simulink model "J2N6S200_simulink_Joint_manipulator"  (R2024a)
settings: Solver=VariableStepAuto  StartTime=0.0  StopTime=2  RelTol=1e-3
undefined symbols (not defined in the file): Sim3dSensor
libraries: sim3dlib x3, vrlib x3, robotcorelib x2, robotmaniplib x2, sim3dcameralib x2, visionsinks x2, robotsim3dlib x1, pycoexlib x1, dspvision x1
settings Model: Creator=abiro  LastModifiedBy=abiro

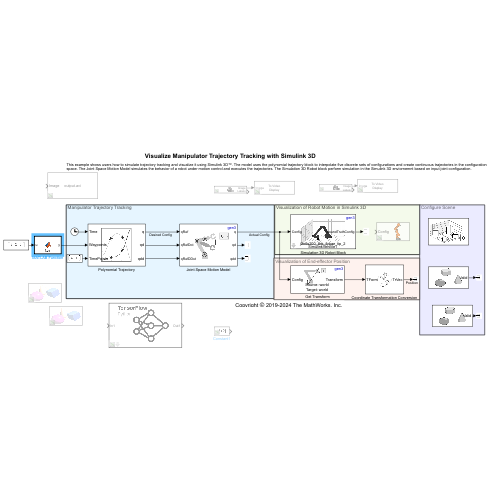
[thumbnail: Simulink's stored preview of the top-level diagram]
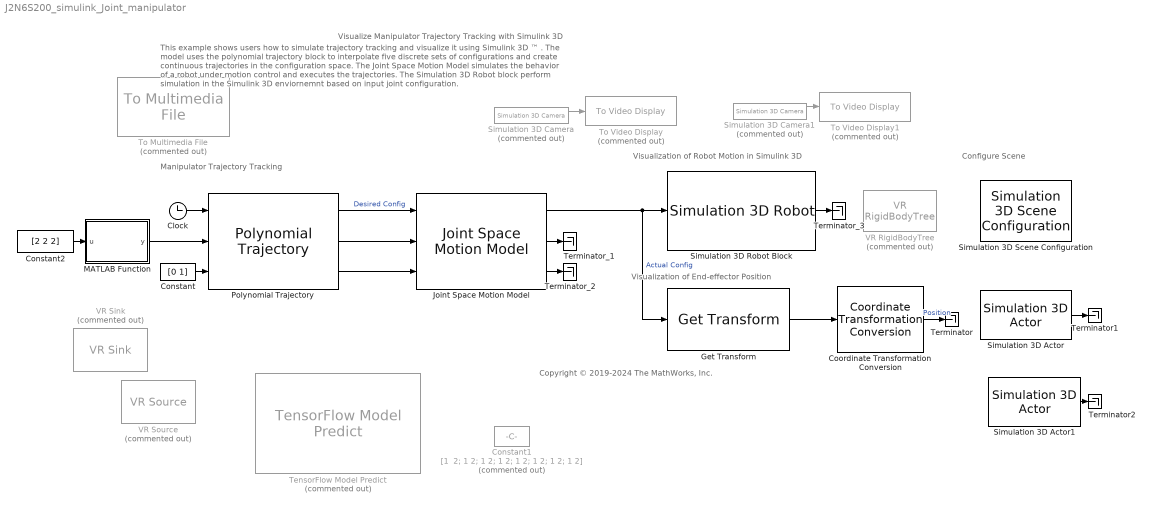
== system J2N6S200_simulink_Joint_manipulator ==
  note: Visualize Manipulator Trajectory Tracking with Simulink 3D
  note: Visualization of Robot Motion in Simulink 3D
  note: This example shows users how to simulate trajectory tracking and visualize it using Simulink 3D ™ . The model uses the polynomial trajectory block to interpolate five discrete sets of configurations and create continuous trajectories in the configuration space. The Joint Space Motion Model simulates the behavior of a robot under motion control and executes the trajectories. The Simulation 3D Robot block perform simulation in the Simulink 3D enviornemnt based on input joint configuration.
  note: Configure Scene
  note: Copyright © 2019-2024 The MathWorks, Inc.
  note: Visualization of End-effector Position
  note: Manipulator Trajectory Tracking
  Clock : Clock
  Constant : Constant  Value=[0 1]  VectorParams1D=off
  Constant1 : Constant  Commented=on  Value="[1  2; 1 2; 1 2; 1 2; 1 2; 1 2; 1 2; 1 2]"  VectorParams1D=off
  Constant2 : Constant  Value=[2 2 2]  VectorParams1D=off
  Coordinate Transformation Conversion : robotcorelib/Coordinate Transformation Conversion  InputRepresentation=Homogeneous Transformation  InputEulerSequence=ZYX  ShowTrVecInputPort=on  OutputRepresentation=Translation Vector  OutputEulerSequence=ZYX  ShowTrVecOutputPort=on  SimulateUsing=Interpreted execution
  Get Transform : robotmaniplib/Get Transform  RigidBodyTree=gen3  SourceBody=world  TargetBody=world  SimulateUsing=Interpreted execution
  Joint Space Motion Model : robotmaniplib/Joint Space Motion Model  RigidBodyTree=gen3  MotionType=Computed Torque Control  ProportionalGain=100  DerivativeGain=10  ErrorDynamicsSpecification=Damping Ratio / Natural Frequency  DampingRatio=1  NaturalFrequency=10  SettlingTime=0.59  Overshoot=0  ShowExternalForcePort=off  InitConfig=0  InitJointVel=0  SimulateUsing=Interpreted execution
  MATLAB Function : MATLAB Function  TreatAsAtomicUnit=on
  Polynomial Trajectory : robotcorelib/Polynomial Trajectory  WaypointSource=External  Waypoints=.75*pi*rand(8,2) - .375*pi  TimePoints=[ 0, 1]  TimeInterval=[ 1, 4 ]  Method=Cubic Polynomial  ParameterSource=Internal  VelocityBoundaryCondition=zeros( 8, 2 )  AccelerationBoundaryCondition=zeros( 2, 5 )  SimulateUsing=Interpreted execution
  Simulation 3D Actor : sim3dlib/Simulation 3D Actor  Priority=1  ActorName=Sim3dActor1  ParentName=Scene Origin  Operation=Create at setup  InitScriptText=|  SampleTime=-1  Translation=single([0 0 0])  Rotation=single([0 0 0])  Scale=single([1 1 1])  aMode=5  ActorTag=Sim3dActor1  ActorType=Sim3dActor  ID=1
      | % Reserved keywords:
      | % - Actor : handle to this actor object
      | % - World : handle to the world object
      | 
      | % Examples:
      | 
      | % Create a primitive geometry (optional)
      | Actor.createShape('box', [10 10 0.1]);
      | 
      | % Initialize values (optional)
      | Actor.Scale = 1;
      | Actor.Color = [0.2 0.2 0.2];
  Simulation 3D Actor1 : sim3dlib/Simulation 3D Actor  Priority=1  ActorName=Sim3dActor2  ParentName=Scene Origin  Operation=Create at setup  InitScriptText=|  SampleTime=-1  Translation=single([0 1 2])  Rotation=single([0 0 0])  Scale=single([1 1 1])  aMode=5  ActorTag=Sim3dActor2  ActorType=Sim3dActor  ID=2
      | % Reserved keywords:
      | % - Actor : handle to this actor object
      | % - World : handle to the world object
      | 
      | % Examples:
      | 
      | % Create a primitive geometry (optional)
      | Actor.createShape('box', [0.2 0.2 0.2]);
      | 
      | % Initialize values (optional)
      | Actor.Scale = 1;
      | Actor.Color = [0.2 0.2 0.2];
  Simulation 3D Camera : sim3dcameralib/Simulation 3D Camera  Priority=1  Commented=on  sensorTag=Sim3dSensor�  sensorId=1  sensorName=Sim3dSensor�  vehTagList={'Scene Origin';'Sim3dActor1';'SimulinkVehicle1'}  vehTag=Sim3dActor1  mountLoc=Origin  offsetFlag=on  tmountOffset=[-3.5, -1, 1]  extTmount=off  rmountOffset=[0, 0, 0]  extRmount=off  FocalLength=[1109, 1109]  OpticalCenter=[640, 360]  ImageSize=[720, 1280]  RadialDistortion=[0, 0]  TangentialDistortion=[0, 0]  SensorSkew=0  DepthOutportEnabled=off  SemanticOutportEnabled=on  TransformOutportEnabled=off  SampleTime=-1  mountPoint=[-3.5 1 1]  mountOrientation=[0 0 0]  aMode=6  ID=1
      settings: LibrarySourceBlock=robotsim3dlib/Simulation 3D Camera
  Simulation 3D Camera1 : sim3dcameralib/Simulation 3D Camera  Priority=1  Commented=on  sensorTag=Sim3dSensor�  sensorId=2  sensorName=Sim3dSensor�  vehTagList={'Scene Origin';'Sim3dActor1';'SimulinkVehicle1'}  vehTag=Sim3dActor1  mountLoc=Origin  offsetFlag=on  tmountOffset=[-3.5, 1, 1]  extTmount=off  rmountOffset=[0, 0, 0]  extRmount=off  FocalLength=[1109, 1109]  OpticalCenter=[640, 360]  ImageSize=[720, 1280]  RadialDistortion=[0, 0]  TangentialDistortion=[0, 0]  SensorSkew=0  DepthOutportEnabled=off  SemanticOutportEnabled=on  TransformOutportEnabled=off  SampleTime=-1  mountPoint=[-3.5 -1 1]  mountOrientation=[0 0 0]  aMode=6  ID=2
      settings: LibrarySourceBlock=robotsim3dlib/Simulation 3D Camera
  Simulation 3D Robot Block : robotsim3dlib/Simulation 3D Robot  actorInputType=RigidBodyTree Object  RigidBodyTree=gen3  ActorName=SimulinkVehicle1  existActorChekBox=off  initialTrans=[0 0 0]  initialRot=[0 0 0]  initialConfig="[0      3.1416      3.1416           0           0           0           0           0]"  EndEffector=j2n6s200_link_finger_tip_2  eeOffsetInpChekBox=off  eeTargetTrans=[0 0 0]  eeTargetRot=[0 0 0]  enableRegionGraspChekBox=off  regionGraspInpChekBox=off  eeTargTransDiff=[0.2 0.2 0.2]  eeTargRotDiff=[0 0 0]  inpConfEnbVal=on  inpGraspEnbVal=off  inpTransEnbVal=off  outConfEnbVal=on  outGraspEnbVal=off  outTransEnbVal=off  SampleTime=0.02  ActorType=SimulinkVehicle  ID=1  aMode=6  ActorTag=SimulinkVehicle1  Mesh=RigidBodyTree
  Simulation 3D Scene Configuration : sim3dlib/Simulation 3D Scene Configuration  Priority=0  ProjectFormat=Default Scenes  SceneDesc=Empty scene  ProjectName=C:\Program Files\MATLAB\R2024a\toolbox\shared\sim3d_projects\automotive_project_windows\UE\WindowsNoEditor\VehicleSimulation.exe  ScenePath=/Game/Maps/EmptyScene  EnableOpenDRIVE=off  vehTagList={'Custom';'Scene Origin';'Sim3dActor1';'SimulinkVehicle1'}  vehTag=Scene Origin  FreeCameraInitialTranslation=[0, 0, 0]  FreeCameraDefaultInitialTranslation=[-6, 0, 2]  FreeCameraInitialRotation=[0, 0, 0]  FreeCameraDefaultInitialRotation=[0, -15, 0]  OpVisEn=off  Ts=0.02  EnableWindow=on  EnableRemoteAccess=off  EnableWeather=off  SunAzimuth=90  SunAltitude=40.0  EnableGeospatialSun=off  Latitude=0  Longitude=0  Date=2023-01-01  Time=10:30:00  GeoTimeZone=-5.0  SunDaylightSaving=off  wind=1  clouds=10  EnableVolumetricClouds=off  CloudCoverage=0  CloudAltitude=6  fog=0  rain=0  RaindropsEffect=off  SnowDensity=0  EnableGeospatial=off  UseTrueOrigin=off  OriginHeight=200  OriginLatitude=40.744652  OriginLongitude=-73.988864  MapStyle=Aerial  AdditionalAssetIDs=[]  UseAdvancedSunSky=off  SolarTime=11  TimeZone=-5  Day=21  Month=9  Year=2022  UseDaylightSavingTime=on  DSTStartDay=10  DSTStartMonth=3  DSTEndDay=3  DSTEndMonth=11  DSTSwitchHour=2  sensorTag=MainCamera1  sensorId=1  sensorName=MainCamera1  mountLoc=Origin  offsetFlag=off  tmountOffset=[0, 0, 0]  rmountOffset=[0, 0, 0]  HorizontalResolution=1280  VerticalResolution=720  HorizontalFOV=60  mountPoint=[0 0 0]  mountOrientation=[0 0 0]  aMode=6  ID=1  GeoTrigger=Inactive
      settings: LibrarySourceBlock=robotsim3dlib/Simulation 3D Scene Configuration
  TensorFlow Model Predict : pycoexlib/TensorFlow Model Predict  Commented=on  ModelFile=untitled  InputTable={'In1','float32','','inherit'}  OutputTable={'Out1','',''}  SampleTime=-1  InputDatatypes=float32  InputNumDims=inherit  InputPermutations=[]  OutputPermutations=[]  PythonCoexecutionBlockType=TensorFlowModelBlock  VariableOutputMaxSizes=[]
  Terminator : Terminator
  Terminator1 : Terminator
  Terminator2 : Terminator
  Terminator_1 : Terminator
  Terminator_2 : Terminator
  Terminator_3 : Terminator
  To Multimedia File : dspvision/To Multimedia File  Commented=on  outputFilename=output.avi  streamSelection=Video only  videoCompressor=None (uncompressed)  audioCompressor=None (uncompressed)  imagePorts=One multidimensional signal  fileType=AVI  audioDatatype=Determine from input data type  fourcc=RGB  audioBitRate=128  audioQuality=75  videoQuality=75  mj2000CompFactor=10
      settings: LibrarySourceBlock=visionsinks/To Multimedia File
  To Video Display : visionsinks/To Video Display  Commented=on  windowSizeMode=Normal  openAtMdlStart=on  fullScreen=off  videoWindowX=536805376  videoWindowY=536805376  saveWindowSize=off  videoWindowWidth=2147483647  videoWindowHeight=2147483647  inputColorFormat=RGB  inputType=Obsolete  imagePorts=One multidimensional signal  OutputDevice=On-screen video monitor  dataOrg=Column-major  isWindowOpen=off
  To Video Display1 : visionsinks/To Video Display  Commented=on  windowSizeMode=Normal  openAtMdlStart=on  fullScreen=off  videoWindowX=536805376  videoWindowY=536805376  saveWindowSize=off  videoWindowWidth=2147483647  videoWindowHeight=2147483647  inputColorFormat=RGB  inputType=Obsolete  imagePorts=One multidimensional signal  OutputDevice=On-screen video monitor  dataOrg=Column-major  isWindowOpen=off
  VR RigidBodyTree : vrlib/VR RigidBodyTree  Commented=on  RBT=[]  useRBT=off  Ts=-1  ForceViewerOpen=off
  VR Sink : vrlib/VR Sink  Commented=on  InstantiateOnLoad=on  SampleTime=0.1  ViewEnable=on  RemoteChange=off  RemoteView=on  AutoView=off  VideoDimensions=[]  AllowVariableSize=off  FigureProperties=[]
  VR Source : vrlib/VR Source  Commented=on  InstantiateOnLoad=on  SampleTime=0.1  ViewEnable=on  RemoteChange=off  RemoteView=on  AutoView=off  VideoDimensions=[]  AllowVariableSize=off  FigureProperties=[]
  wires:
  Joint Space Motion Model/2 -> Terminator_1/1
  Joint Space Motion Model/1 -> Simulation 3D Robot Block/1, Get Transform/1  "Actual Config"
  Coordinate Transformation Conversion/1 -> Terminator/1  "Position"
  Joint Space Motion Model/3 -> Terminator_2/1
  Simulation 3D Actor/1 -> Terminator1/1
  Get Transform/1 -> Coordinate Transformation Conversion/1
  Polynomial Trajectory/3 -> Joint Space Motion Model/3
  Clock/1 -> Polynomial Trajectory/1
  Polynomial Trajectory/1 -> Joint Space Motion Model/1  "Desired Config"
  Polynomial Trajectory/2 -> Joint Space Motion Model/2
  Simulation 3D Camera/1 -> To Video Display/1
  Simulation 3D Camera1/1 -> To Video Display1/1
  Simulation 3D Robot Block/1 -> Terminator_3/1
  Simulation 3D Actor1/1 -> Terminator2/1
  Constant/1 -> Polynomial Trajectory/3
  Constant2/1 -> MATLAB Function/1(u)
  MATLAB Function/1(y) -> Polynomial Trajectory/2

== matlab function J2N6S200_simulink_Joint_manipulator/MATLAB Function ==
  data: u input; y output
function y = fcn(u)

y = zeros(8,2);%similar to variable declaration
waypoints = zeros(3,2);%similar to variable declaration

gen3 = loadrobot("kinovaJacoJ2N6S200");%loads as a rigid body tree
gen3.DataFormat = 'column';%setting DataFormat = 'column' ensures that any joint configuration or velocity data you pass to functions like getTransform are represented as column vectors, rather than rows.
q_home = [0 135 -90 0 -130 0 90 90]'*pi/180;%convert to radians always
%%%%%%%%%%%%%%%%%%%%%
%NOTE: The last two are the grippers, they are right now in full grip
%position.
%%%%%%%%%%%%%%%%%%%%%
eeName = 'j2n6s200_end_effector';%this is part of the robot, you can list this with some function
T_home = getTransform(gen3, q_home, eeName);%transform = getTransform(robot,configuration,bodyname) computes the transform that converts points in the bodyname frame to the robot base frame, using the specified robot configuration.

waypoints(:,1) = T_home(1:3,4);%both are columns
T_home(1:4,4) =  [0;0;0;1];%for some reason the the transformation blocks last column is converted to this
%implies row 1 to 4, column 4, we can also simply use : instead of 1:4 in this case
%if you want to replace a column then its " = [ 0 0 0 1 ]"

%every ; marks the end of a row
waypoints(:,2) = u';%LHS is a column, RHS is a row vector so its transposed
orientations = [pi/2    0   pi/2;% I think this is for the end effector wrt ground, but in the simulation there was full down orientation too
                pi/2    0   pi/2]';


ik = inverseKinematics('RigidBodyTree',gen3);%an object associated with gen3
ikWeights = [1 1 1 1 1 1];%The vector [1 1 1 1 1 1] defines the relative importance (or weights) for each element in the 
% target pose: [x, y, z, roll, pitch, yaw]. The weights indicate how strictly the solver should aim to meet each of the pose requirements.
% In this case, all pose elements are equally weighted.
ikInitGuess = q_home';%the single quotes represents transpose and the home position is taking as a initial guess for non linear optimisation
ikInitGuess(ikInitGuess > pi) = ikInitGuess(ikInitGuess > pi) - 2*pi;%bringing any values above +pi to below
ikInitGuess(ikInitGuess < -pi) = ikInitGuess(ikInitGuess < -pi) + 2*pi;%bringing any values below -pi to below


includeOrientation = false; %each column in waypoints represents a coordinate (end effector wants to reach)
numWaypoints = size(waypoints,2);%2 here represents column
numJoints = 8;
jointWaypoints = zeros(numJoints,numWaypoints);

for idx = 1:numWaypoints % a for loop
    if includeOrientation
        tgtPose = trvec2tform(waypoints(:,idx)') * eul2tform(orientations(:,idx)');
    else
        tgtPose = trvec2tform(waypoints(:,idx)') * eul2tform([pi/2 0 pi/2]); %#ok<UNRCH> this is the default
    end
    [config,info] = ik(eeName,tgtPose,ikWeights',ikInitGuess');
    jointWaypoints(:,idx) = config';%will be 8 rows and 2 columns in the end
end

y = jointWaypoints;
